simulink model "Oren_Sim"  (R2020b)
settings: Solver=VariableStepAuto  StartTime=0.0  StopTime=Params.tf  FixedStep=1e-2  RelTol=1e-8  AbsTol=1e-8
undefined symbols (not defined in the file or in its folder): Params, rad, s
libraries: aerolibconvert2 x1, simulink_extras x1, sharedutil x1
settings Model: Creator=orena  LastModifiedBy=orena

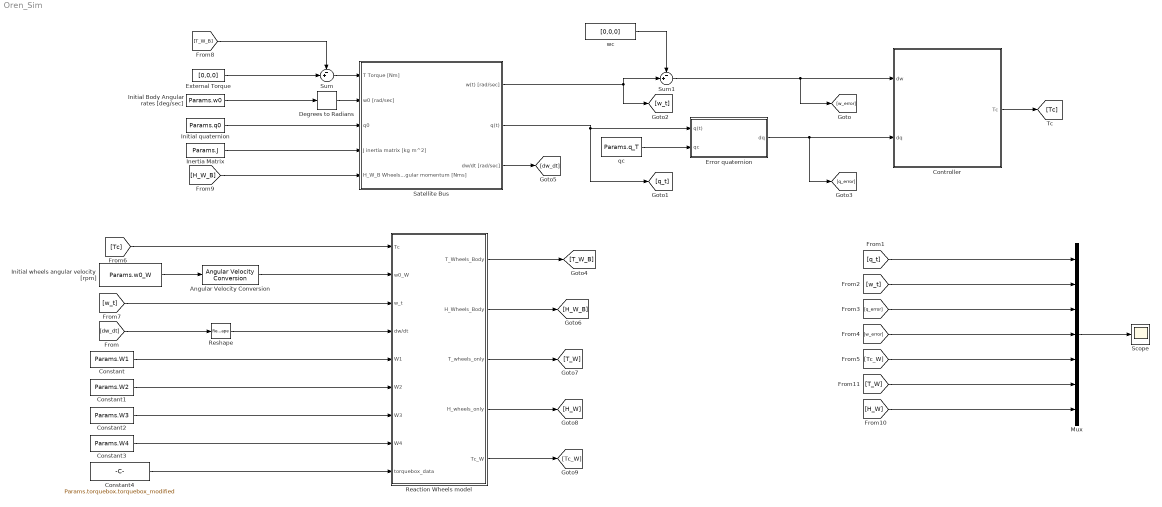
== system Oren_Sim ==
  Angular Velocity Conversion : aerolibconvert2/Angular Velocity Conversion  IU=rpm  OU=rad/s
  Constant : Constant  Value=Params.W1
  Constant1 : Constant  Value=Params.W2
  Constant2 : Constant  Value=Params.W3
  Constant3 : Constant  Value=Params.W4
  Constant4 : Constant  Value=Params.torquebox.torquebox_modified
  Controller : Subsystem
  Degrees to Radians : simulink_extras/Transformations/Degrees to Radians
  Error quaternion : Subsystem
  External Torque : Constant  Value=[0,0,0]
  Inertia Matrix : Constant  Value=Params.J
  Initial Body Angular rates [deg/sec] : Constant  Value=Params.w0
  Initial quaternion : Constant  Value=Params.q0
  Initial wheels angular velocity [rpm] : Constant  Value=Params.w0_W
  Mux : Mux  Inputs=7
  Reaction Wheels model : Subsystem
  Reshape : Reshape  OutputDimensionality=Column vector (2-D)
  Satellite Bus : Subsystem
  Scope : Scope
  Sum : Sum  Inputs=-+|
  Sum1 : Sum  Inputs=-+|
  qc : Constant  Value=Params.q_T
  wc : Constant  Value=[0,0,0]
  wires:
  Initial Body Angular rates [deg/sec]/1 -> Degrees to Radians/1
  External Torque/1 -> Sum/2
  Controller/1(Tc) -> [Tc]
  [T_W_B] -> Sum/1
  wc/1 -> Sum1/1
  Sum/1 -> Satellite Bus/1(T Torque [Nm])
  Degrees to Radians/1 -> Satellite Bus/2(w0 [rad/sec])
  Initial quaternion/1 -> Satellite Bus/3(q0)
  Inertia Matrix/1 -> Satellite Bus/4(J inertia matrix [kg m^2])
  qc/1 -> Error quaternion/2(qc)
  Satellite Bus/2(q(t)) -> [q_t], Error quaternion/1(q(t))
  Error quaternion/1(dq) -> [q_error], Controller/2(dq)
  Satellite Bus/1(w(t) [rad/sec]) -> Sum1/2, [w_t]
  Sum1/1 -> [w_error], Controller/1(dw)
  Mux/1 -> Scope/1
  [q_t] -> Mux/1
  [w_t] -> Mux/2
  [q_error] -> Mux/3
  [w_error] -> Mux/4
  [Tc_W] -> Mux/5
  Initial wheels angular velocity [rpm]/1 -> Angular Velocity Conversion/1
  Angular Velocity Conversion/1 -> Reaction Wheels model/2(w0_W)
  [Tc] -> Reaction Wheels model/1(Tc)
  [w_t] -> Reaction Wheels model/3(w_t)
  Reaction Wheels model/1(T_Wheels_Body) -> [T_W_B]
  Satellite Bus/3(dw/dt [rad/sec]) -> [dw_dt]
  [dw_dt] -> Reshape/1
  Constant/1 -> Reaction Wheels model/5(W1)
  Constant1/1 -> Reaction Wheels model/6(W2)
  Constant2/1 -> Reaction Wheels model/7(W3)
  Constant3/1 -> Reaction Wheels model/8(W4)
  Reaction Wheels model/2(H_Wheels_Body) -> [H_W_B]
  Reaction Wheels model/3(T_wheels_only) -> [T_W]
  Reaction Wheels model/4(H_wheels_only) -> [H_W]
  [H_W_B] -> Satellite Bus/5(H_W_B Wheels angular momentum [Nms])
  [H_W] -> Mux/7
  [T_W] -> Mux/6
  Constant4/1 -> Reaction Wheels model/9(torquebox_data)
  Reshape/1 -> Reaction Wheels model/4(dw/dt)
  Reaction Wheels model/5(Tc_W) -> [Tc_W]

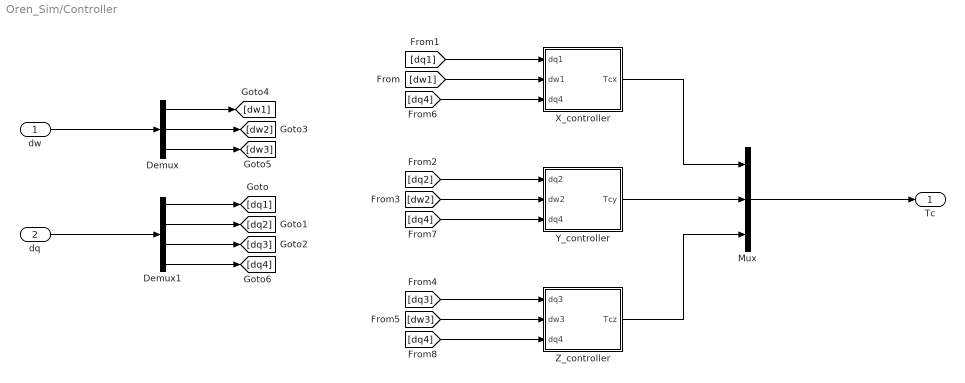
== system Oren_Sim/Controller ==
  dw : Inport
  dq : Inport  Port=2
  Demux : Demux  Outputs=3
  Demux1 : Demux
  Mux : Mux  Inputs=3
  X_controller : Subsystem
  Y_controller : Subsystem
  Z_controller : Subsystem
  Tc : Outport
  wires:
  Demux/1 -> [dw1]
  [dw2] -> Y_controller/2(dw2)
  [dq1] -> X_controller/1(dq1)
  [dq3] -> Z_controller/1(dq3)
  Demux/2 -> [dw2]
  Demux/3 -> [dw3]
  [dw3] -> Z_controller/2(dw3)
  Demux1/3 -> [dq3]
  Demux1/1 -> [dq1]
  Demux1/2 -> [dq2]
  [dq2] -> Y_controller/1(dq2)
  dw/1 -> Demux/1
  [dw1] -> X_controller/2(dw1)
  Y_controller/1(Tcy) -> Mux/2
  X_controller/1(Tcx) -> Mux/1
  Z_controller/1(Tcz) -> Mux/3
  dq/1 -> Demux1/1
  Demux1/4 -> [dq4]
  [dq4] -> X_controller/3(dq4)
  [dq4] -> Y_controller/3(dq4)
  [dq4] -> Z_controller/3(dq4)
  Mux/1 -> Tc/1

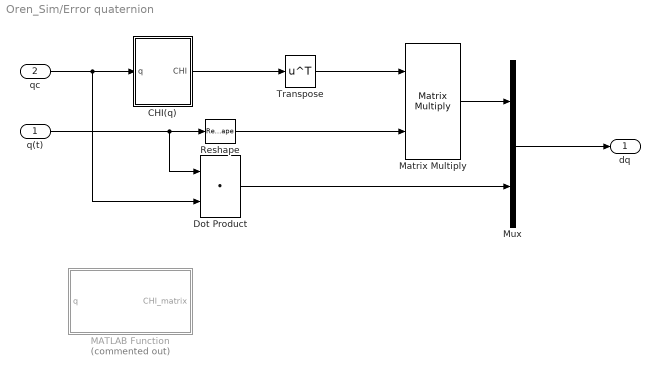
== system Oren_Sim/Error quaternion ==
  q(t) : Inport
  qc : Inport  Port=2
  CHI(q) : Subsystem
  Dot Product : DotProduct  InputSameDT=on  OutDataTypeStr=Inherit: Inherit via internal rule
  MATLAB Function : MATLAB Function  Commented=on  TreatAsAtomicUnit=on
  Matrix Multiply : Product  Multiplication=Matrix(*)
  Mux : Mux  Inputs=2
  Reshape : Reshape  OutputDimensionality=Column vector (2-D)
  Transpose : Math  Operator=transpose  SaturateOnIntegerOverflow=on
  dq : Outport
  wires:
  q(t)/1 -> Dot Product/1, Reshape/1
  Reshape/1 -> Matrix Multiply/2
  CHI(q)/1(CHI) -> Transpose/1
  qc/1 -> Dot Product/2, CHI(q)/1(q)
  Transpose/1 -> Matrix Multiply/1
  Matrix Multiply/1 -> Mux/1
  Mux/1 -> dq/1
  Dot Product/1 -> Mux/2

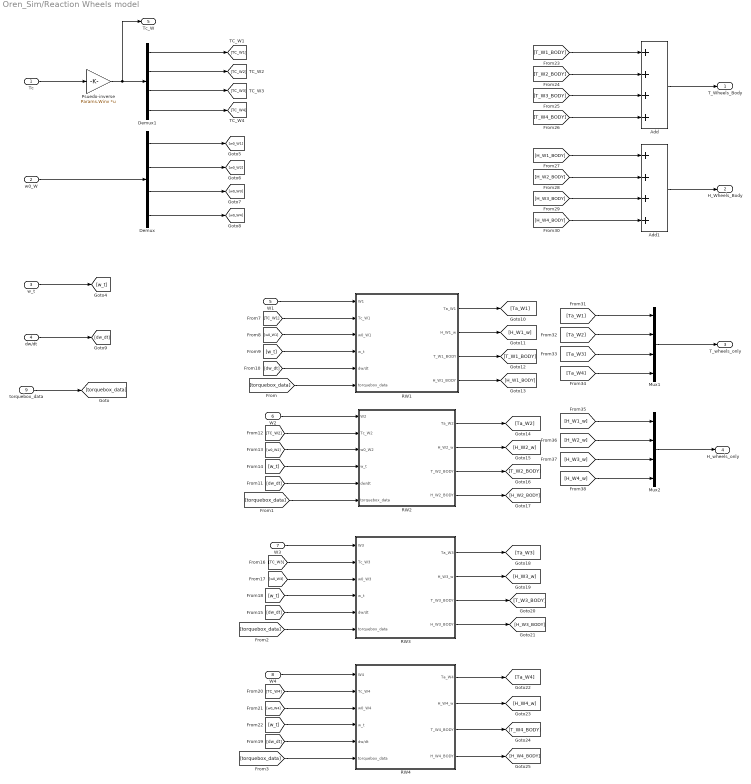
== system Oren_Sim/Reaction Wheels model ==
  Tc : Inport
  w0_W : Inport  Port=2
  w_t : Inport  Port=3
  dw/dt : Inport  Port=4
  W1 : Inport  Port=5
  W2 : Inport  Port=6
  W3 : Inport  Port=7
  W4 : Inport  Port=8
  torquebox_data : Inport  Port=9
  Add : Sum  Inputs=++++
  Add1 : Sum  Inputs=++++
  Demux : Demux
  Demux1 : Demux
  Mux1 : Mux
  Mux2 : Mux
  Psuedo-inverse : Gain  Gain=Params.Winv  Multiplication=Matrix(K*u) (u vector)
  RW1 : Subsystem
  RW2 : Subsystem
  RW3 : Subsystem
  RW4 : Subsystem
  T_Wheels_Body : Outport
  H_Wheels_Body : Outport  Port=2
  T_wheels_only : Outport  Port=3
  H_wheels_only : Outport  Port=4
  Tc_W : Outport  Port=5
  wires:
  RW2/3(T_W2_BODY) -> [T_W2_BODY]
  [H_W1_BODY] -> Add1/1
  W2/1 -> RW2/1(W2)
  Add1/1 -> H_Wheels_Body/1
  [TC_W1] -> RW1/2(Tc_W1)
  Demux/3 -> [w0_W3]
  Mux2/1 -> H_wheels_only/1
  dw/dt/1 -> [dw_dt]
  Tc/1 -> Psuedo-inverse/1
  RW2/2(H_W2_w) -> [H_W2_w]
  W3/1 -> RW3/1(W3)
  w0_W/1 -> Demux/1
  [H_W2_BODY] -> Add1/2
  Psuedo-inverse/1 -> Tc_W/1, Demux1/1
  W1/1 -> RW1/1(W1)
  [w_t] -> RW1/4(w_t)
  [w_t] -> RW4/4(w_t)
  [TC_W2] -> RW2/2(Tc_W2)
  Demux1/4 -> [TC_W4]
  RW3/3(T_W3_BODY) -> [T_W3_BODY]
  RW1/4(H_W1_BODY) -> [H_W1_BODY]
  [T_W2_BODY] -> Add/2
  RW2/4(H_W2_BODY) -> [H_W2_BODY]
  [Ta_W2] -> Mux1/2
  [dw_dt] -> RW3/5(dw/dt)
  [w_t] -> RW2/4(w_t)
  [H_W4_BODY] -> Add1/4
  RW4/3(T_W4_BODY) -> [T_W4_BODY]
  [H_W4_w] -> Mux2/4
  RW3/2(H_W3_w) -> [H_W3_w]
  RW1/3(T_W1_BODY) -> [T_W1_BODY]
  RW4/4(H_W4_BODY) -> [H_W4_BODY]
  [dw_dt] -> RW1/5(dw/dt)
  RW3/4(H_W3_BODY) -> [H_W3_BODY]
  [Ta_W4] -> Mux1/4
  RW2/1(Ta_W2) -> [Ta_W2]
  Demux1/1 -> [TC_W1]
  [Ta_W1] -> Mux1/1
  w_t/1 -> [w_t]
  Mux1/1 -> T_wheels_only/1
  RW4/2(H_W4_w) -> [H_W4_w]
  [T_W4_BODY] -> Add/4
  Demux/4 -> [w0_W4]
  [w0_W2] -> RW2/3(w0_W2)
  [dw_dt] -> RW4/5(dw/dt)
  [TC_W3] -> RW3/2(Tc_W3)
  Demux1/3 -> [TC_W3]
  [dw_dt] -> RW2/5(dw/dt)
  W4/1 -> RW4/1(W4)
  [H_W3_w] -> Mux2/3
  RW1/2(H_W1_w) -> [H_W1_w]
  [w_t] -> RW3/4(w_t)
  [TC_W4] -> RW4/2(Tc_W4)
  [w0_W1] -> RW1/3(w0_W1)
  RW1/1(Ta_W1) -> [Ta_W1]
  Demux/1 -> [w0_W1]
  RW3/1(Ta_W3) -> [Ta_W3]
  Demux1/2 -> [TC_W2]
  Demux/2 -> [w0_W2]
  [T_W3_BODY] -> Add/3
  [H_W1_w] -> Mux2/1
  Add/1 -> T_Wheels_Body/1
  [w0_W3] -> RW3/3(w0_W3)
  [w0_W4] -> RW4/3(w0_W4)
  RW4/1(Ta_W4) -> [Ta_W4]
  [H_W2_w] -> Mux2/2
  [H_W3_BODY] -> Add1/3
  [T_W1_BODY] -> Add/1
  [Ta_W3] -> Mux1/3
  torquebox_data/1 -> [torquebox_data]
  [torquebox_data] -> RW1/6(torquebox_data)
  [torquebox_data] -> RW2/6(torquebox_data)
  [torquebox_data] -> RW3/6(torquebox_data)
  [torquebox_data] -> RW4/6(torquebox_data)

== system Oren_Sim/Satellite Bus ==
  T Torque [Nm] : Inport
  w0 [rad/sec] : Inport  Port=2
  q0 : Inport  Port=3
  J inertia matrix [kg m^2] : Inport  Port=4
  H_W_B Wheels angular momentum [Nms] : Inport  Port=5
  Satellite Dynamics : Subsystem
  Satellite Kinematics : Subsystem
  w(t) [rad/sec] : Outport
  q(t) : Outport  Port=2
  dw/dt [rad/sec] : Outport  Port=3
  wires:
  q0/1 -> Satellite Kinematics/2(q0)
  Satellite Kinematics/1(q(t)) -> q(t)/1
  J inertia matrix [kg m^2]/1 -> Satellite Dynamics/3(J inertia matrix [kg m^2])
  w0 [rad/sec]/1 -> Satellite Dynamics/2(w0 [rad/sec])
  Satellite Dynamics/1(w(t) [rad/sec]) -> Satellite Kinematics/1(w(t) [rad/sec]), w(t) [rad/sec]/1
  T Torque [Nm]/1 -> Satellite Dynamics/1(T Torque [Nm])
  Satellite Dynamics/2(dw/dt [rad/sec^2]) -> dw/dt [rad/sec]/1
  H_W_B Wheels angular momentum [Nms]/1 -> Satellite Dynamics/4(H_W_B Wheels angular momentum [Nms])

== system Oren_Sim/Controller/X_controller ==
  dq1 : Inport
  dw1 : Inport  Port=2
  dq4 : Inport  Port=3
  Gain : Gain  Gain=Params.gains.kdx
  Gain1 : Gain  Gain=Params.gains.kpx
  Product : Product
  Sign : Signum
  Sum2 : Sum  Inputs=+|+
  Tcx : Outport
  wires:
  Sum2/1 -> Tcx/1
  dq1/1 -> Gain1/1
  dw1/1 -> Gain/1
  Gain/1 -> Sum2/2
  dq4/1 -> Sign/1
  Sign/1 -> Product/1
  Gain1/1 -> Product/2
  Product/1 -> Sum2/1

== system Oren_Sim/Controller/Y_controller ==
  dq2 : Inport
  dw2 : Inport  Port=2
  dq4 : Inport  Port=3
  Gain2 : Gain  Gain=Params.gains.kpy
  Gain3 : Gain  Gain=Params.gains.kdy
  Product : Product
  Sign : Signum
  Sum3 : Sum  Inputs=+|+
  Tcy : Outport
  wires:
  dq2/1 -> Gain2/1
  Gain3/1 -> Sum3/2
  Sum3/1 -> Tcy/1
  dw2/1 -> Gain3/1
  dq4/1 -> Sign/1
  Sign/1 -> Product/1
  Gain2/1 -> Product/2
  Product/1 -> Sum3/1

== system Oren_Sim/Controller/Z_controller ==
  dq3 : Inport
  dw3 : Inport  Port=2
  dq4 : Inport  Port=3
  Gain4 : Gain  Gain=Params.gains.kpz
  Gain5 : Gain  Gain=Params.gains.kdz
  Product : Product
  Sign : Signum
  Sum4 : Sum  Inputs=+|+
  Tcz : Outport
  wires:
  Sum4/1 -> Tcz/1
  dw3/1 -> Gain5/1
  Gain5/1 -> Sum4/2
  dq3/1 -> Gain4/1
  dq4/1 -> Sign/1
  Sign/1 -> Product/1
  Gain4/1 -> Product/2
  Product/1 -> Sum4/1

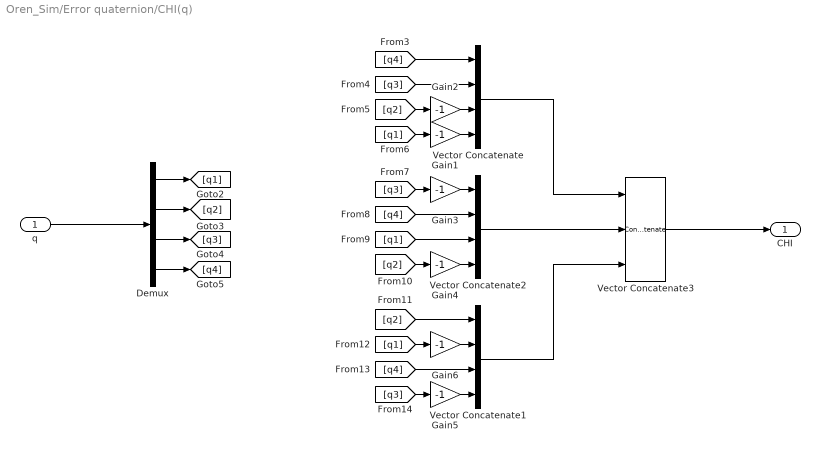
== system Oren_Sim/Error quaternion/CHI(q) ==
  q : Inport
  Demux : Demux
  Gain{1..6} (6 alike) : Gain  Gain=-1
  Vector Concatenate : Concatenate  NumInputs=4
  Vector Concatenate1 : Concatenate  NumInputs=4
  Vector Concatenate2 : Concatenate  NumInputs=4
  Vector Concatenate3 : Concatenate  NumInputs=3  Mode=Multidimensional array  ConcatenateDimension=2
  CHI : Outport
  wires:
  [q1] -> Vector Concatenate2/3
  [q3] -> Gain5/1
  Vector Concatenate3/1 -> CHI/1
  Vector Concatenate/1 -> Vector Concatenate3/1
  Vector Concatenate2/1 -> Vector Concatenate3/2
  q/1 -> Demux/1
  [q3] -> Gain3/1
  Gain3/1 -> Vector Concatenate2/1
  [q3] -> Vector Concatenate/2
  [q4] -> Vector Concatenate1/3
  [q1] -> Gain1/1
  Demux/2 -> [q2]
  Gain1/1 -> Vector Concatenate/4
  Demux/3 -> [q3]
  [q4] -> Vector Concatenate/1
  [q4] -> Vector Concatenate2/2
  Gain4/1 -> Vector Concatenate2/4
  [q2] -> Vector Concatenate1/1
  Demux/1 -> [q1]
  [q1] -> Gain6/1
  Gain6/1 -> Vector Concatenate1/2
  [q2] -> Gain2/1
  [q2] -> Gain4/1
  Gain2/1 -> Vector Concatenate/3
  Vector Concatenate1/1 -> Vector Concatenate3/3
  Demux/4 -> [q4]
  Gain5/1 -> Vector Concatenate1/4

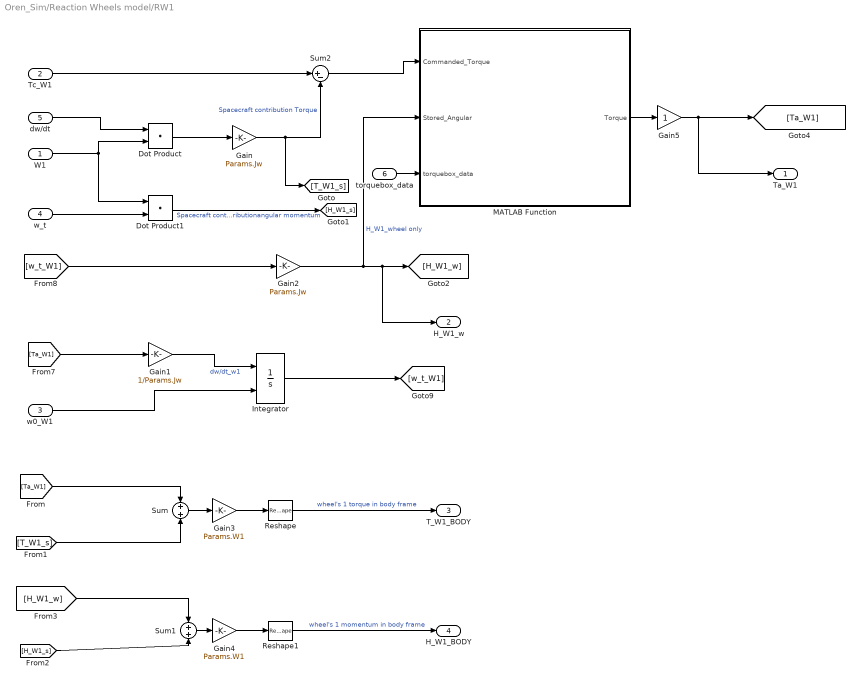
== system Oren_Sim/Reaction Wheels model/RW1 ==
  W1 : Inport
  Tc_W1 : Inport  Port=2
  w0_W1 : Inport  Port=3
  w_t : Inport  Port=4
  dw/dt : Inport  Port=5
  torquebox_data : Inport  Port=6
  Dot Product : DotProduct  InputSameDT=on  OutDataTypeStr=Inherit: Inherit via internal rule
  Dot Product1 : DotProduct  InputSameDT=on  OutDataTypeStr=Inherit: Inherit via internal rule
  Gain : Gain  Gain=Params.Jw
  Gain1 : Gain  Gain=1/Params.Jw
  Gain2 : Gain  Gain=Params.Jw
  Gain3 : Gain  Gain=Params.W1
  Gain4 : Gain  Gain=Params.W1
  Gain5 : Gain
  Integrator : Integrator  InitialConditionSource=external
  MATLAB Function : MATLAB Function  TreatAsAtomicUnit=on
  Reshape : Reshape  OutputDimensionality=Column vector (2-D)
  Reshape1 : Reshape  OutputDimensionality=Column vector (2-D)
  Sum : Sum  Inputs=+|+
  Sum1 : Sum  Inputs=+|+
  Sum2 : Sum  Inputs=|+-
  Ta_W1 : Outport
  H_W1_w : Outport  Port=2
  T_W1_BODY : Outport  Port=3
  H_W1_BODY : Outport  Port=4
  wires:
  Tc_W1/1 -> Sum2/1
  Gain/1 -> Sum2/2, [T_W1_s]  "Spacecraft contribution Torque"
  dw/dt/1 -> Dot Product/1
  w0_W1/1 -> Integrator/2
  Sum2/1 -> MATLAB Function/1(Commanded_Torque)
  W1/1 -> Dot Product1/1, Dot Product/2
  Dot Product/1 -> Gain/1
  Gain2/1 -> H_W1_w/1, [H_W1_w], MATLAB Function/2(Stored_Angular)  "H_W1_wheel only"
  [Ta_W1] -> Gain1/1
  Integrator/1 -> [w_t_W1]
  Gain1/1 -> Integrator/1  "dw/dt_w1"
  [w_t_W1] -> Gain2/1
  w_t/1 -> Dot Product1/2
  Dot Product1/1 -> [H_W1_s]  "Spacecraft contributionangular momentum"
  [Ta_W1] -> Sum/1
  [T_W1_s] -> Sum/2
  Sum/1 -> Gain3/1
  [H_W1_s] -> Sum1/2
  [H_W1_w] -> Sum1/1
  Sum1/1 -> Gain4/1
  Gain3/1 -> Reshape/1
  Gain4/1 -> Reshape1/1
  Reshape/1 -> T_W1_BODY/1  "wheel's 1 torque in body frame"
  Reshape1/1 -> H_W1_BODY/1  "wheel's 1 momentum in body frame"
  torquebox_data/1 -> MATLAB Function/3(torquebox_data)
  MATLAB Function/1(Torque) -> Gain5/1
  Gain5/1 -> Ta_W1/1, [Ta_W1]

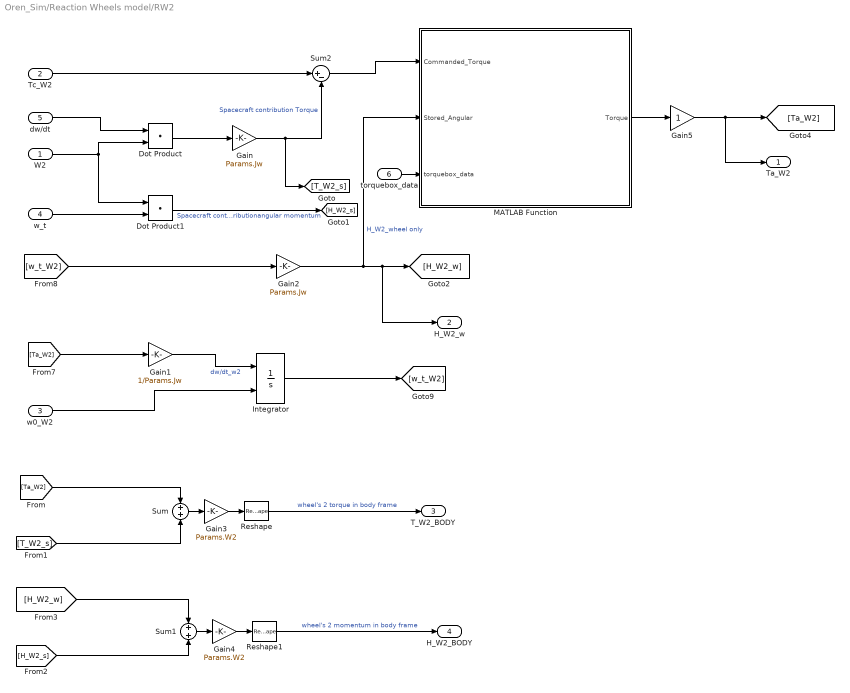
== system Oren_Sim/Reaction Wheels model/RW2 ==
  W2 : Inport
  Tc_W2 : Inport  Port=2
  w0_W2 : Inport  Port=3
  w_t : Inport  Port=4
  dw/dt : Inport  Port=5
  torquebox_data : Inport  Port=6
  Dot Product : DotProduct  InputSameDT=on  OutDataTypeStr=Inherit: Inherit via internal rule
  Dot Product1 : DotProduct  InputSameDT=on  OutDataTypeStr=Inherit: Inherit via internal rule
  Gain : Gain  Gain=Params.Jw
  Gain1 : Gain  Gain=1/Params.Jw
  Gain2 : Gain  Gain=Params.Jw
  Gain3 : Gain  Gain=Params.W2
  Gain4 : Gain  Gain=Params.W2
  Gain5 : Gain
  Integrator : Integrator  InitialConditionSource=external
  MATLAB Function : MATLAB Function  TreatAsAtomicUnit=on
  Reshape : Reshape  OutputDimensionality=Column vector (2-D)
  Reshape1 : Reshape  OutputDimensionality=Column vector (2-D)
  Sum : Sum  Inputs=+|+
  Sum1 : Sum  Inputs=+|+
  Sum2 : Sum  Inputs=|+-
  Ta_W2 : Outport
  H_W2_w : Outport  Port=2
  T_W2_BODY : Outport  Port=3
  H_W2_BODY : Outport  Port=4
  wires:
  Gain4/1 -> Reshape1/1
  Gain3/1 -> Reshape/1
  Sum1/1 -> Gain4/1
  [H_W2_w] -> Sum1/1
  [H_W2_s] -> Sum1/2
  Sum/1 -> Gain3/1
  [T_W2_s] -> Sum/2
  [Ta_W2] -> Sum/1
  Dot Product1/1 -> [H_W2_s]  "Spacecraft contributionangular momentum"
  w_t/1 -> Dot Product1/2
  [w_t_W2] -> Gain2/1
  Gain1/1 -> Integrator/1  "dw/dt_w2"
  Integrator/1 -> [w_t_W2]
  [Ta_W2] -> Gain1/1
  Gain2/1 -> MATLAB Function/2(Stored_Angular), [H_W2_w], H_W2_w/1  "H_W2_wheel only"
  Dot Product/1 -> Gain/1
  W2/1 -> Dot Product/2, Dot Product1/1
  Sum2/1 -> MATLAB Function/1(Commanded_Torque)
  w0_W2/1 -> Integrator/2
  dw/dt/1 -> Dot Product/1
  Gain/1 -> [T_W2_s], Sum2/2  "Spacecraft contribution Torque"
  Tc_W2/1 -> Sum2/1
  Reshape/1 -> T_W2_BODY/1  "wheel's 2 torque in body frame"
  Reshape1/1 -> H_W2_BODY/1  "wheel's 2 momentum in body frame"
  torquebox_data/1 -> MATLAB Function/3(torquebox_data)
  MATLAB Function/1(Torque) -> Gain5/1
  Gain5/1 -> Ta_W2/1, [Ta_W2]

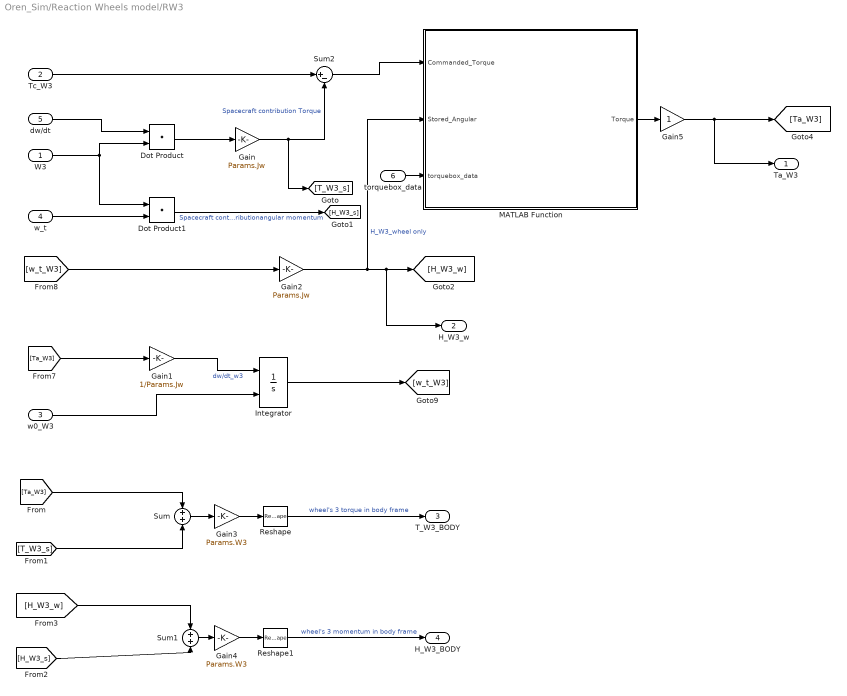
== system Oren_Sim/Reaction Wheels model/RW3 ==
  W3 : Inport
  Tc_W3 : Inport  Port=2
  w0_W3 : Inport  Port=3
  w_t : Inport  Port=4
  dw/dt : Inport  Port=5
  torquebox_data : Inport  Port=6
  Dot Product : DotProduct  InputSameDT=on  OutDataTypeStr=Inherit: Inherit via internal rule
  Dot Product1 : DotProduct  InputSameDT=on  OutDataTypeStr=Inherit: Inherit via internal rule
  Gain : Gain  Gain=Params.Jw
  Gain1 : Gain  Gain=1/Params.Jw
  Gain2 : Gain  Gain=Params.Jw
  Gain3 : Gain  Gain=Params.W3
  Gain4 : Gain  Gain=Params.W3
  Gain5 : Gain
  Integrator : Integrator  InitialConditionSource=external
  MATLAB Function : MATLAB Function  TreatAsAtomicUnit=on
  Reshape : Reshape  OutputDimensionality=Column vector (2-D)
  Reshape1 : Reshape  OutputDimensionality=Column vector (2-D)
  Sum : Sum  Inputs=+|+
  Sum1 : Sum  Inputs=+|+
  Sum2 : Sum  Inputs=|+-
  Ta_W3 : Outport
  H_W3_w : Outport  Port=2
  T_W3_BODY : Outport  Port=3
  H_W3_BODY : Outport  Port=4
  wires:
  Tc_W3/1 -> Sum2/1
  Gain/1 -> Sum2/2, [T_W3_s]  "Spacecraft contribution Torque"
  dw/dt/1 -> Dot Product/1
  w0_W3/1 -> Integrator/2
  Sum2/1 -> MATLAB Function/1(Commanded_Torque)
  W3/1 -> Dot Product1/1, Dot Product/2
  Dot Product/1 -> Gain/1
  Gain2/1 -> H_W3_w/1, [H_W3_w], MATLAB Function/2(Stored_Angular)  "H_W3_wheel only"
  [Ta_W3] -> Gain1/1
  Integrator/1 -> [w_t_W3]
  Gain1/1 -> Integrator/1  "dw/dt_w3"
  [w_t_W3] -> Gain2/1
  w_t/1 -> Dot Product1/2
  Dot Product1/1 -> [H_W3_s]  "Spacecraft contributionangular momentum"
  [Ta_W3] -> Sum/1
  [T_W3_s] -> Sum/2
  Sum/1 -> Gain3/1
  [H_W3_s] -> Sum1/2
  [H_W3_w] -> Sum1/1
  Sum1/1 -> Gain4/1
  Gain3/1 -> Reshape/1
  Gain4/1 -> Reshape1/1
  Reshape/1 -> T_W3_BODY/1  "wheel's 3 torque in body frame"
  Reshape1/1 -> H_W3_BODY/1  "wheel's 3 momentum in body frame"
  torquebox_data/1 -> MATLAB Function/3(torquebox_data)
  MATLAB Function/1(Torque) -> Gain5/1
  Gain5/1 -> Ta_W3/1, [Ta_W3]

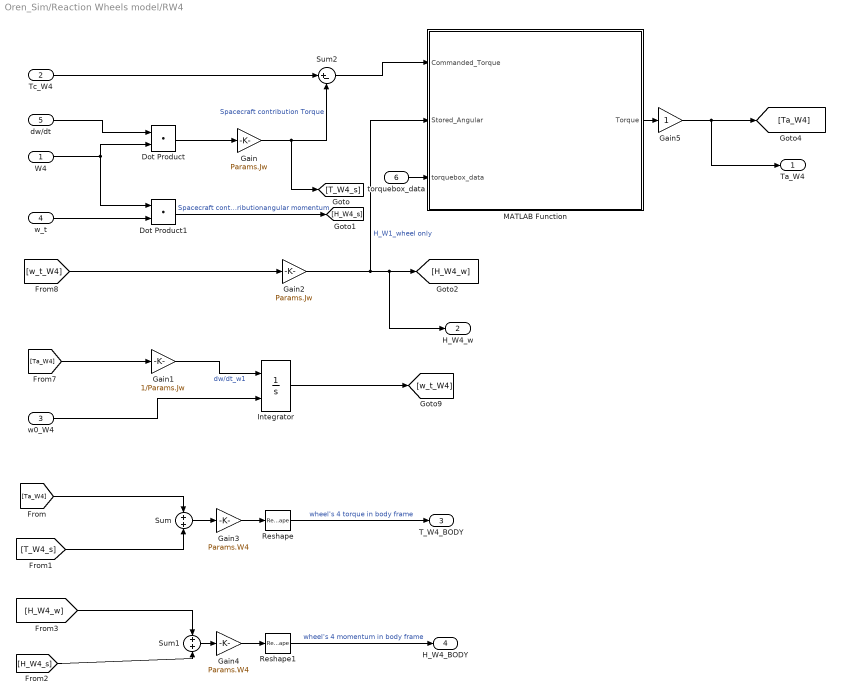
== system Oren_Sim/Reaction Wheels model/RW4 ==
  W4 : Inport
  Tc_W4 : Inport  Port=2
  w0_W4 : Inport  Port=3
  w_t : Inport  Port=4
  dw/dt : Inport  Port=5
  torquebox_data : Inport  Port=6
  Dot Product : DotProduct  InputSameDT=on  OutDataTypeStr=Inherit: Inherit via internal rule
  Dot Product1 : DotProduct  InputSameDT=on  OutDataTypeStr=Inherit: Inherit via internal rule
  Gain : Gain  Gain=Params.Jw
  Gain1 : Gain  Gain=1/Params.Jw
  Gain2 : Gain  Gain=Params.Jw
  Gain3 : Gain  Gain=Params.W4
  Gain4 : Gain  Gain=Params.W4
  Gain5 : Gain
  Integrator : Integrator  InitialConditionSource=external
  MATLAB Function : MATLAB Function  TreatAsAtomicUnit=on
  Reshape : Reshape  OutputDimensionality=Column vector (2-D)
  Reshape1 : Reshape  OutputDimensionality=Column vector (2-D)
  Sum : Sum  Inputs=+|+
  Sum1 : Sum  Inputs=+|+
  Sum2 : Sum  Inputs=|+-
  Ta_W4 : Outport
  H_W4_w : Outport  Port=2
  T_W4_BODY : Outport  Port=3
  H_W4_BODY : Outport  Port=4
  wires:
  Gain4/1 -> Reshape1/1
  Gain3/1 -> Reshape/1
  Sum1/1 -> Gain4/1
  [H_W4_w] -> Sum1/1
  [H_W4_s] -> Sum1/2
  Sum/1 -> Gain3/1
  [T_W4_s] -> Sum/2
  [Ta_W4] -> Sum/1
  Dot Product1/1 -> [H_W4_s]  "Spacecraft contributionangular momentum"
  w_t/1 -> Dot Product1/2
  [w_t_W4] -> Gain2/1
  Gain1/1 -> Integrator/1  "dw/dt_w1"
  Integrator/1 -> [w_t_W4]
  [Ta_W4] -> Gain1/1
  Gain2/1 -> MATLAB Function/2(Stored_Angular), [H_W4_w], H_W4_w/1  "H_W1_wheel only"
  Dot Product/1 -> Gain/1
  W4/1 -> Dot Product/2, Dot Product1/1
  Sum2/1 -> MATLAB Function/1(Commanded_Torque)
  w0_W4/1 -> Integrator/2
  dw/dt/1 -> Dot Product/1
  Gain/1 -> [T_W4_s], Sum2/2  "Spacecraft contribution Torque"
  Tc_W4/1 -> Sum2/1
  Reshape/1 -> T_W4_BODY/1  "wheel's 4 torque in body frame"
  Reshape1/1 -> H_W4_BODY/1  "wheel's 4 momentum in body frame"
  torquebox_data/1 -> MATLAB Function/3(torquebox_data)
  MATLAB Function/1(Torque) -> Gain5/1
  Gain5/1 -> Ta_W4/1, [Ta_W4]

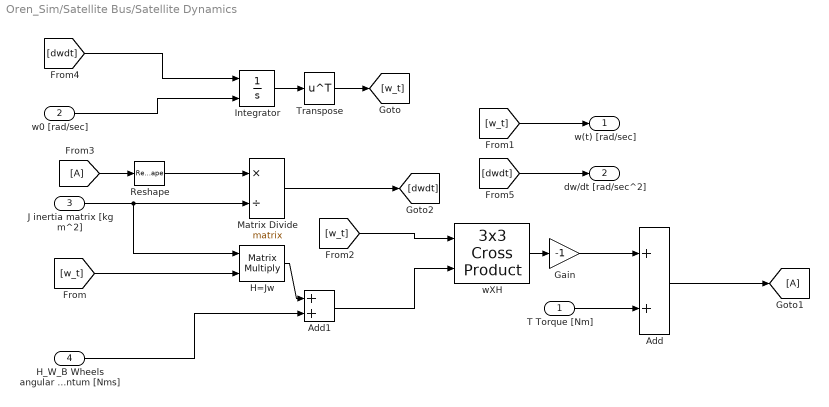
== system Oren_Sim/Satellite Bus/Satellite Dynamics ==
  T Torque [Nm] : Inport
  w0 [rad/sec] : Inport  Port=2
  J inertia matrix [kg m^2] : Inport  Port=3
  H_W_B Wheels angular momentum [Nms] : Inport  Port=4
  Add : Sum
  Add1 : Sum
  Gain : Gain  Gain=-1
  H=Jw : Product  Multiplication=Matrix(*)
  Integrator : Integrator  InitialConditionSource=external
  Matrix Divide : Product  Inputs=*/  Multiplication=Matrix(*)
  Reshape : Reshape  OutputDimensionality=Row vector (2-D)
  Transpose : Math  Operator=transpose  SaturateOnIntegerOverflow=on
  wXH : sharedutil/3x3 Cross Product  aMode=aMode
      settings: SourceProductBaseCode=AE,PW,MT,UV,VE,VP
  w(t) [rad/sec] : Outport
  dw/dt [rad/sec^2] : Outport  Port=2
  wires:
  T Torque [Nm]/1 -> Add/2
  w0 [rad/sec]/1 -> Integrator/2
  Gain/1 -> Add/1
  [w_t] -> w(t) [rad/sec]/1
  J inertia matrix [kg m^2]/1 -> Matrix Divide/2, H=Jw/1
  [dwdt] -> Integrator/1
  wXH/1 -> Gain/1
  [w_t] -> wXH/1
  [A] -> Reshape/1
  Matrix Divide/1 -> [dwdt]
  [w_t] -> H=Jw/2
  Integrator/1 -> Transpose/1
  Transpose/1 -> [w_t]
  [dwdt] -> dw/dt [rad/sec^2]/1
  H_W_B Wheels angular momentum [Nms]/1 -> Add1/2
  Add/1 -> [A]
  H=Jw/1 -> Add1/1
  Add1/1 -> wXH/2
  Reshape/1 -> Matrix Divide/1

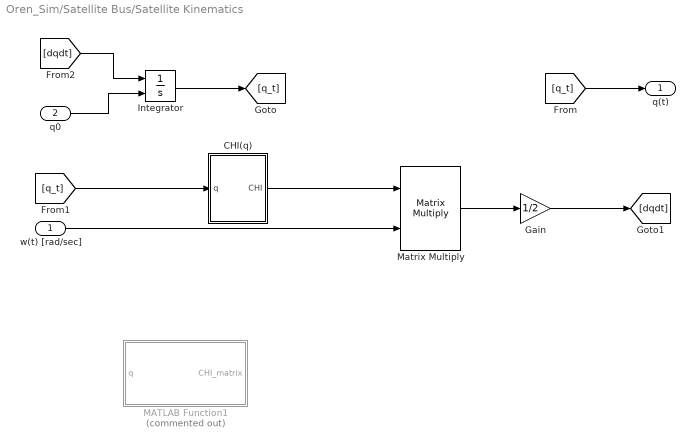
== system Oren_Sim/Satellite Bus/Satellite Kinematics ==
  w(t) [rad/sec] : Inport
  q0 : Inport  Port=2
  CHI(q) : Subsystem
  Gain : Gain  Gain=1/2
  Integrator : Integrator  InitialConditionSource=external
  MATLAB Function1 : MATLAB Function  Commented=on  TreatAsAtomicUnit=on
  Matrix Multiply : Product  Multiplication=Matrix(*)
  q(t) : Outport
  wires:
  [dqdt] -> Integrator/1
  [q_t] -> q(t)/1
  Gain/1 -> [dqdt]
  Integrator/1 -> [q_t]
  Matrix Multiply/1 -> Gain/1
  q0/1 -> Integrator/2
  w(t) [rad/sec]/1 -> Matrix Multiply/2
  CHI(q)/1(CHI) -> Matrix Multiply/1
  [q_t] -> CHI(q)/1(q)

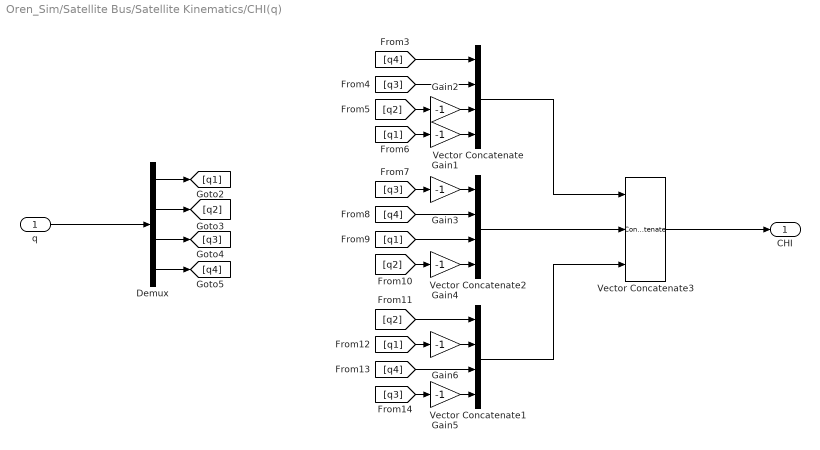
== system Oren_Sim/Satellite Bus/Satellite Kinematics/CHI(q) ==
  q : Inport
  Demux : Demux
  Gain{1..6} (6 alike) : Gain  Gain=-1
  Vector Concatenate : Concatenate  NumInputs=4
  Vector Concatenate1 : Concatenate  NumInputs=4
  Vector Concatenate2 : Concatenate  NumInputs=4
  Vector Concatenate3 : Concatenate  NumInputs=3  Mode=Multidimensional array  ConcatenateDimension=2
  CHI : Outport
  wires:
  [q1] -> Vector Concatenate2/3
  [q3] -> Gain5/1
  Vector Concatenate3/1 -> CHI/1
  Vector Concatenate/1 -> Vector Concatenate3/1
  Vector Concatenate2/1 -> Vector Concatenate3/2
  q/1 -> Demux/1
  [q3] -> Gain3/1
  Gain3/1 -> Vector Concatenate2/1
  [q3] -> Vector Concatenate/2
  [q4] -> Vector Concatenate1/3
  [q1] -> Gain1/1
  Demux/2 -> [q2]
  Gain1/1 -> Vector Concatenate/4
  Demux/3 -> [q3]
  [q4] -> Vector Concatenate/1
  [q4] -> Vector Concatenate2/2
  Gain4/1 -> Vector Concatenate2/4
  [q2] -> Vector Concatenate1/1
  Demux/1 -> [q1]
  [q1] -> Gain6/1
  Gain6/1 -> Vector Concatenate1/2
  [q2] -> Gain2/1
  [q2] -> Gain4/1
  Gain2/1 -> Vector Concatenate/3
  Vector Concatenate1/1 -> Vector Concatenate3/3
  Demux/4 -> [q4]
  Gain5/1 -> Vector Concatenate1/4

== matlab function Oren_Sim/Reaction Wheels model/RW2/MATLAB Function ==
  data: Commanded_Torque input; Torque output; Stored_Angular input; torquebox_data input
function Torque = RW_Torque(Commanded_Torque,Stored_Angular,torquebox_data)
Torque = Allowed_torque(Commanded_Torque, Stored_Angular, torquebox_data);

== matlab function Oren_Sim/Satellite Bus/Satellite Kinematics/MATLAB Function1 ==
  data: q input; CHI_matrix output
function CHI_matrix = CHI(q)

CHI_matrix = [q(4),-q(3),q(2);...
              q(3),q(4),-q(1);...
              -q(2),q(1),q(4);...
             -q(1),-q(2),-q(3)];

== matlab function Oren_Sim/Reaction Wheels model/RW3/MATLAB Function ==
  data: Commanded_Torque input; Torque output; Stored_Angular input; torquebox_data input
function Torque = RW_Torque(Commanded_Torque,Stored_Angular,torquebox_data)
Torque = Allowed_torque(Commanded_Torque, Stored_Angular, torquebox_data);

== matlab function Oren_Sim/Reaction Wheels model/RW4/MATLAB Function ==
  data: Commanded_Torque input; Torque output; Stored_Angular input; torquebox_data input
function Torque = RW_Torque(Commanded_Torque,Stored_Angular,torquebox_data)
Torque = Allowed_torque(Commanded_Torque, Stored_Angular, torquebox_data);

== matlab function Oren_Sim/Reaction Wheels model/RW1/MATLAB Function ==
  data: Commanded_Torque input; Torque output; Stored_Angular input; torquebox_data input
function Torque = RW_Torque(Commanded_Torque,Stored_Angular,torquebox_data)
Torque = Allowed_torque(Commanded_Torque, Stored_Angular, torquebox_data);

== matlab function Oren_Sim/Error quaternion/MATLAB Function ==
  data: q input; CHI_matrix output
function CHI_matrix = CHI(q)

CHI_matrix = [q(4),-q(3),q(2);...
              q(3),q(4),-q(1);...
              -q(2),q(1),q(4);...
             -q(1),-q(2),-q(3)];
